simulink model "drugi"  (R2024b)
settings: Solver=VariableStepAuto  StartTime=0.0  StopTime=10.0  RelTol=1e-3
settings Model: Creator=DT User  LastModifiedBy=DT User

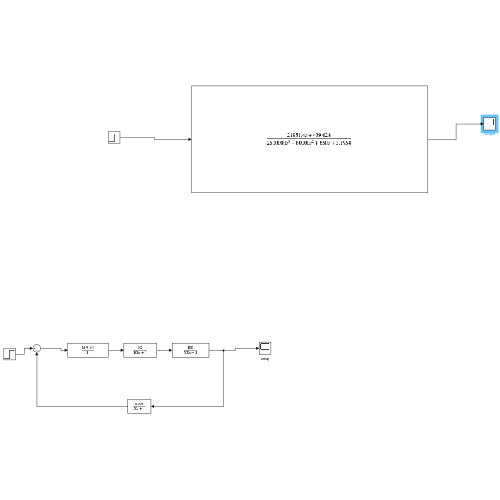
[thumbnail: Simulink's stored preview of the top-level diagram]
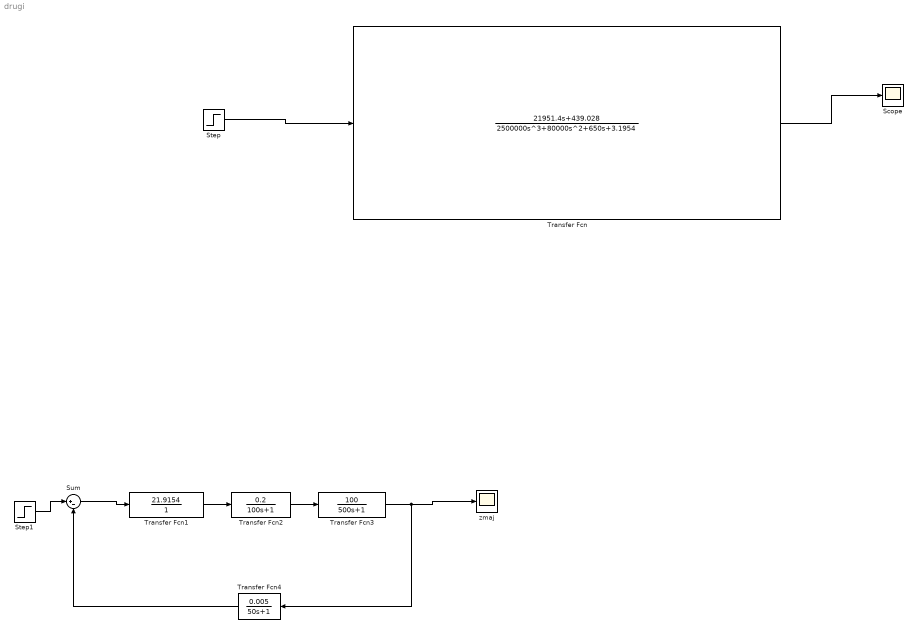
== system drugi ==
  Scope : Scope
  Step : Step  SampleTime=0
  Step1 : Step  SampleTime=0
  Sum : Sum  Inputs=|+-
  Transfer Fcn : TransferFcn  Numerator=[21951.4 439.028]  Denominator=[2500000 80000 650 3.1954]
  Transfer Fcn1 : TransferFcn  Numerator=[21.9154]  Denominator=1
  Transfer Fcn2 : TransferFcn  Numerator=[0.2]  Denominator=[100 1]
  Transfer Fcn3 : TransferFcn  Numerator=[100]  Denominator=[500 1]
  Transfer Fcn4 : TransferFcn  Numerator=[0.005]  Denominator=[50 1]
  zmaj : Scope
  wires:
  Step/1 -> Transfer Fcn/1
  Transfer Fcn/1 -> Scope/1
  Transfer Fcn3/1 -> Transfer Fcn4/1, zmaj/1
  Transfer Fcn2/1 -> Transfer Fcn3/1
  Transfer Fcn1/1 -> Transfer Fcn2/1
  Sum/1 -> Transfer Fcn1/1
  Transfer Fcn4/1 -> Sum/2
  Step1/1 -> Sum/1
